simulink model "sampleModel155"  (R2021b)
settings: Solver=VariableStepAuto  StartTime=0.0  StopTime=10.0  RelTol=1e-3
undefined symbols (not defined in the file or in its folder): DiscIntNeverNeededParam, Newton, Raphson
libraries: simulink x4, slpidlib x1
settings Model: Creator=user  LastModifiedBy=user

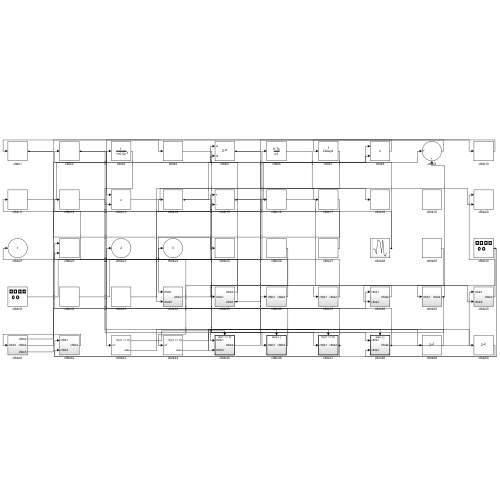
[thumbnail: Simulink's stored preview of the top-level diagram]
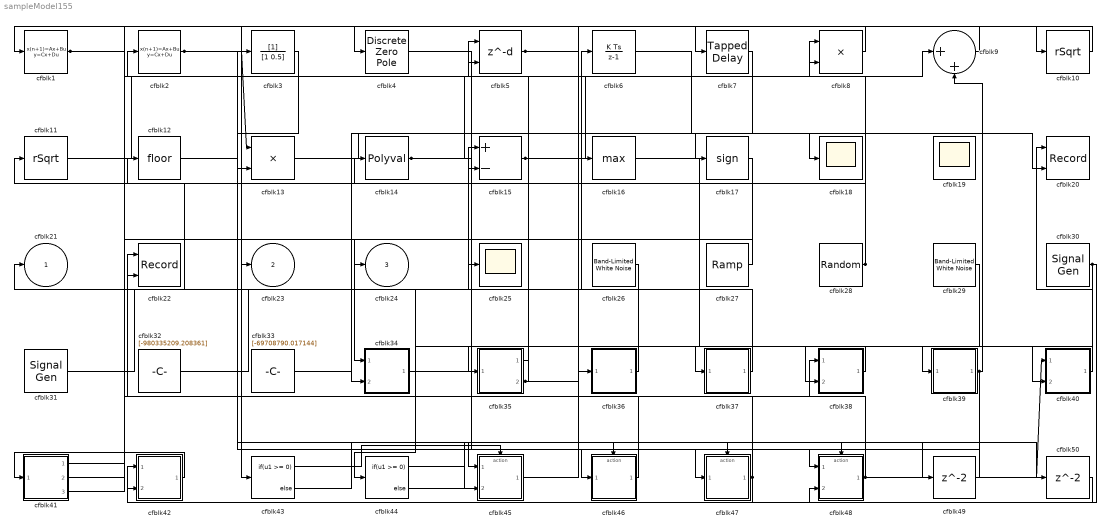
== system sampleModel155 ==
  cfblk1 : DiscreteStateSpace
  cfblk10 : Sqrt  Operator=rSqrt  AlgorithmType=Newton-Raphson  SaturateOnIntegerOverflow=on
  cfblk11 : Sqrt  Operator=rSqrt  AlgorithmType=Newton-Raphson  SaturateOnIntegerOverflow=on
  cfblk12 : Rounding
  cfblk13 : Product  Inputs=**
  cfblk14 : Polyval  Coefs=[ +2.081618890e-019, -1.441693666e-014, +4.719686976e-010, -8.536869453e-006, +1.621573104e-001, -8.087801117e+001 ]
  cfblk15 : Sum  Inputs=+-
  cfblk16 : MinMax  Function=max
  cfblk17 : Signum
  cfblk18 : Scope
  cfblk19 : Scope
      settings: Floating=on
  cfblk2 : DiscreteStateSpace
  cfblk20 : Record  FileSettingsInternal="{\"entries\":[{\"content\":{\"excelSettings\":{\"content\":{},\"type\":\"Streamout.ExcelSettings\"}},\"type\":\"Streamout.FileSettingStorage\",\"uuid\":\"c6a0a69c-cb25-483f-9436-b518442c183b\"}],\"packageUris\":[\"http://schema.mathworks.com/mf0/streamout_blocks/R2020a\"],\"version\":\"1.0\"}"  Layout=[1 1]  SignalsInternal="{\"entries\":[{\"content\":{\"signals\":[{\"content\":{\"blockPath\":[\"sampleModel155/cfblk20\"],\"channel\":[],\"dimensions\":[1],\"domain\":\"sampleModel155/cfblk20\",\"lineColor\":\"#a2142f\",\"plots\":[1],\"port\":1,\"sid\":[\"\"],\"signalID\":5829,\"signalName\":\"cfblk40\"},\"type\":\"RecordBlkView.Signal\",\"uuid\":\"982e78fb-ecc7-4af2-9bce-bf19e89cf4a4\"},{\"content\":{\"blockPath\":[\"sampleModel155/cfblk20\"],\"channel\":[],\"dimensions\":[1],\"domain\":\"sampleModel155/cfblk20\",\"lineColor\":\"#139fff\",\"plots\":[1],\"port\":2,\"sid\":[\"\"],\"signalID\":5833,\"signalName\":\"cfblk6\"},\"type\":\"RecordBlkView.Signal\",\"uuid\":\"4fc80603-e495-4758-b370-e399ca86c921\"}]},\"type\":\"RecordBlkView.InputSignals\",\"uuid\":\"2fc9934d-8013-4f67-99c3-7600cfd9b416\"}],\"packageUris\":[\"http://schema.mathworks.com/mf0/streamout_blocks/R2020a\"],\"version\":\"1.0\"}"  VisualizationBindings="{\"xyplotplugin\":{\"info\":[{\"series\":[{\"bindingParametersList\":[{\"parameter\":\"X-Axis\",\"signalID\":5829,\"signalName\":\"cfblk40\"},{\"parameter\":\"Y-Axis\",\"signalID\":5833,\"signalName\":\"cfblk6\"}],\"seriesID\":42704}],\"subplotID\":1}]}}"  CompatibilityTag=XY
  cfblk22 : Record  FileSettingsInternal="{\"entries\":[{\"content\":{\"excelSettings\":{\"content\":{},\"type\":\"Streamout.ExcelSettings\"}},\"type\":\"Streamout.FileSettingStorage\",\"uuid\":\"4d11d9fd-29c9-4ce8-99ba-2382077eddbc\"}],\"packageUris\":[\"http://schema.mathworks.com/mf0/streamout_blocks/R2020a\"],\"version\":\"1.0\"}"  Layout=[1 1]  SignalsInternal="{\"entries\":[{\"content\":{\"signals\":[{\"content\":{\"blockPath\":[\"sampleModel155/cfblk22\"],\"channel\":[],\"dimensions\":[1],\"domain\":\"sampleModel155/cfblk22\",\"lineColor\":\"#a2142f\",\"plots\":[1],\"port\":1,\"sid\":[\"\"],\"signalID\":5837,\"signalName\":\"cfblk35:2\"},\"type\":\"RecordBlkView.Signal\",\"uuid\":\"607973d4-97f1-4e95-a130-668d98db00e6\"},{\"content\":{\"blockPath\":[\"sampleModel155/cfblk22\"],\"channel\":[],\"dimensions\":[1],\"domain\":\"sampleModel155/cfblk22\",\"lineColor\":\"#139fff\",\"plots\":[1],\"port\":2,\"sid\":[\"\"],\"signalID\":5841,\"signalName\":\"cfblk48\"},\"type\":\"RecordBlkView.Signal\",\"uuid\":\"b323fbb3-43dc-4456-bc21-4a787fbff72d\"}]},\"type\":\"RecordBlkView.InputSignals\",\"uuid\":\"74f477da-4040-45bf-b858-66ad6525a84b\"}],\"packageUris\":[\"http://schema.mathworks.com/mf0/streamout_blocks/R2020a\"],\"version\":\"1.0\"}"  VisualizationBindings="{\"xyplotplugin\":{\"info\":[{\"series\":[{\"bindingParametersList\":[{\"parameter\":\"X-Axis\",\"signalID\":5837,\"signalName\":\"cfblk35:2\"},{\"parameter\":\"Y-Axis\",\"signalID\":5841,\"signalName\":\"cfblk48\"}],\"seriesID\":8769}],\"subplotID\":1}]}}"  CompatibilityTag=XY
  cfblk25 : Scope
  cfblk26 : simulink/Sources/Band-Limited White Noise  Cov=[6682375464.485454]  Ts=0.1  seed=[5360034971.000000]
  cfblk27 : simulink/Sources/Ramp  slope=[-7060.642561]  start=[21.976533]  InitialOutput=[864381.445498]
  cfblk28 : RandomNumber  Mean=[-62257.725679]  Variance=[20771.732840]  Seed=[583175511.000000]  SampleTime=0.1
  cfblk29 : simulink/Sources/Band-Limited White Noise  Cov=[2781141721.159909]  Ts=0.1  seed=[7793621344.000000]
  cfblk3 : DiscreteFilter  SampleTime=1
  cfblk30 : SignalGenerator  Amplitude=[-532353384.064106]
  cfblk31 : SignalGenerator  WaveForm=sawtooth  Amplitude=[-996285201.899179]  Units=rad/sec
  cfblk32 : Constant  Value=[-980335209.208361]  SampleTime=1
  cfblk33 : Constant  Value=[-69708790.017144]  SampleTime=1
  cfblk34 : Subsystem
  cfblk35 : Subsystem
  cfblk36 : Subsystem
  cfblk37 : Subsystem
  cfblk38 : Subsystem
  cfblk39 : Subsystem
  cfblk4 : DiscreteZeroPole  Poles=[0 0.5]  Gain=1
  cfblk40 : Subsystem
  cfblk41 : Subsystem
  cfblk42 : Subsystem
  cfblk43 : If  IfExpression=u1 >= 0  SampleTime=1
  cfblk44 : If  IfExpression=u1 >= 0  SampleTime=1
  cfblk45 : Subsystem  TreatAsAtomicUnit=on
  cfblk46 : Subsystem  TreatAsAtomicUnit=on
  cfblk47 : Subsystem  TreatAsAtomicUnit=on
  cfblk48 : Subsystem  TreatAsAtomicUnit=on
  cfblk49 : Delay  SampleTime=1
  cfblk5 : Delay  DelayLengthSource=Input port  SampleTime=1
      settings: InputPortMap=u0,p1
  cfblk50 : Delay  SampleTime=1
  cfblk6 : DiscreteIntegrator  ICPrevOutput=DiscIntNeverNeededParam  ICPrevScaledInput=DiscIntNeverNeededParam
  cfblk7 : simulink/Discrete/Tapped Delay  vinit=0.0  samptime=-1  NumDelays=1  DelayOrder=Oldest  includeCurrent=off
  cfblk8 : Product
  cfblk9 : Sum  Inputs=|++
  cfblk21 : Outport
  cfblk23 : Outport  Port=2
  cfblk24 : Outport  Port=3
  wires:
  cfblk4/1 -> cfblk48/1(cfblk1)
  cfblk48/1(cfblk2) -> cfblk40/1(cfblk1), cfblk22/2
  cfblk17/1 -> cfblk34/1(cfblk1)
  cfblk14/1 -> cfblk46/1(cfblk1), cfblk8/2
  cfblk10/1 -> cfblk43/1
  cfblk27/1 -> cfblk11/1
  cfblk29/1 -> cfblk39/1(cfblk1)
  cfblk32/1 -> cfblk15/1
  cfblk28/1 -> cfblk2/1, cfblk14/1
  cfblk45/1(cfblk2) -> cfblk36/1(cfblk1)
  cfblk13/1 -> cfblk18/1
  cfblk34/1(cfblk2) -> cfblk37/1(cfblk1)
  cfblk30/1 -> cfblk42/1(cfblk1), cfblk38/2(cfblk4)
  cfblk26/1 -> cfblk44/1
  cfblk2/1 -> cfblk13/1, cfblk47/1(cfblk1)
  cfblk41/1(cfblk2) -> cfblk5/1
  cfblk46/1(cfblk2) -> cfblk23/1
  cfblk1/1 -> cfblk25/1, cfblk4/1
  cfblk40/1(cfblk2) -> cfblk20/1
  cfblk9/1 -> cfblk7/1
  cfblk6/1 -> cfblk20/2
  cfblk7/1 -> cfblk34/2(cfblk3)
  cfblk31/1 -> cfblk6/1
  cfblk42/1(cfblk2) -> cfblk41/1(cfblk1)
  cfblk3/1 -> cfblk13/2
  cfblk39/1(cfblk2) -> cfblk45/2(cfblk5), cfblk9/2
  cfblk47/1(cfblk2) -> cfblk24/1, cfblk42/2(cfblk3)
  cfblk41/2(cfblk4) -> cfblk38/1(cfblk1)
  cfblk8/1 -> cfblk1/1
  cfblk15/1 -> cfblk9/1, cfblk50/1
  cfblk38/1(cfblk2) -> cfblk35/1(cfblk1)
  cfblk35/1(cfblk2) -> cfblk5/2
  cfblk16/1 -> cfblk40/2(cfblk5)
  cfblk5/1 -> cfblk10/1, cfblk17/1
  cfblk37/1(cfblk2) -> cfblk21/1
  cfblk11/1 -> cfblk3/1
  cfblk35/2(cfblk3) -> cfblk22/1, cfblk8/1
  cfblk41/3(cfblk5) -> cfblk15/2
  cfblk36/1(cfblk2) -> cfblk12/1
  cfblk33/1 -> cfblk16/1
  cfblk43/1 -> cfblk45/Action
  cfblk43/2 -> cfblk46/Action
  cfblk44/1 -> cfblk47/Action
  cfblk44/2 -> cfblk48/Action
  cfblk12/1 -> cfblk49/1
  cfblk49/1 -> cfblk45/1(cfblk1)
  cfblk50/1 -> cfblk48/2(cfblk4)

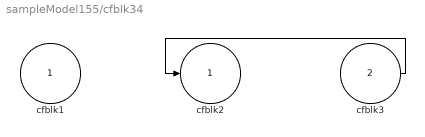
== system sampleModel155/cfblk34 ==
  cfblk1 : Inport
  cfblk3 : Inport  Port=2
  cfblk2 : Outport
  wires:
  cfblk3/1 -> cfblk2/1

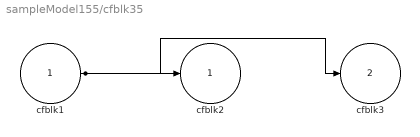
== system sampleModel155/cfblk35 ==
  cfblk1 : Inport
  cfblk2 : Outport
  cfblk3 : Outport  Port=2
  wires:
  cfblk1/1 -> cfblk2/1, cfblk3/1

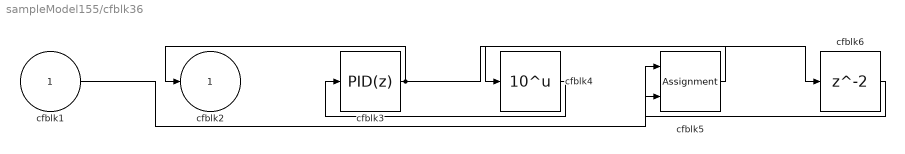
== system sampleModel155/cfblk36 ==
  cfblk1 : Inport
  cfblk3 : slpidlib/PID Controller  Controller=PID  Form=Parallel  TimeDomain=Discrete-time  UseExternalTs=off  SampleTime=1  IntegratorMethod=Forward Euler  FilterMethod=Forward Euler  ControllerParametersSource=internal  P=1  I=1  D=0  UseFilter=on  N=100  TunerSelectOption=Transfer Function Based (PID Tuner App)  InitialConditionSource=internal  InitialConditionForIntegrator=0  InitialConditionForFilter=0  DifferentiatorICPrevScaledInput=0  ExternalReset=none  TrackingMode=off  Kt=1  LimitOutput=off  SatLimitsSource=internal  UpperSaturationLimit=inf  LowerSaturationLimit=-inf  LinearizeAsGain=off  AntiWindupMode=none  Kb=1  POutMin=[]  POutMax=[]  IOutMin=[]  IOutMax=[]  DOutMin=[]  DOutMax=[]  NOutMin=[]  NOutMax=[]  SumOutMin=[]  SumOutMax=[]  SaturationOutMin=[]  SaturationOutMax=[]  PParamMin=[]  PParamMax=[]  IParamMin=[]  IParamMax=[]  DParamMin=[]  DParamMax=[]  NParamMin=[]  NParamMax=[]  KbParamMin=[]  KbParamMax=[]  KtParamMin=[]  KtParamMax=[]  KbOutMin=[]  KbOutMax=[]  KtOutMin=[]  KtOutMax=[]  IntegratorOutMin=[]  IntegratorOutMax=[]  FilterOutMin=[]  FilterOutMax=[]  SumI1OutMin=[]  SumI1OutMax=[]  SumI2OutMin=[]  SumI2OutMax=[]  SumI3OutMin=[]  SumI3OutMax=[]  SumI4OutMin=[]  SumI4OutMax=[]  SumDOutMin=[]  SumDOutMax=[]  DifferentiatorOutMin=[]  DifferentiatorOutMax=[]  FilterDiffOutCoefMin=[]  FilterDiffOutCoefMax=[]  ReciprocalOutMin=[]  ReciprocalOutMax=[]  SumDenOutMin=[]  SumDenOutMax=[]  SumNumOutMin=[]  SumNumOutMax=[]  DivideOutMin=[]  DivideOutMax=[]  UdiffTsProdOutMin=[]  UdiffTsProdOutMax=[]  NTsProdOutMin=[]  NTsProdOutMax=[]  UintegralTsProdOutMin=[]  UintegralTsProdOutMax=[]  UngainTsProdOutMin=[]  UngainTsProdOutMax=[]  IntegratorContinuousStateAttributes=''  IntegratorStateMustResolveToSignalObject=off  IntegratorRTWStateStorageClass=Auto  FilterContinuousStateAttributes=''  FilterStateMustResolveToSignalObject=off  FilterRTWStateStorageClass=Auto  ParallelPVariant=InternalParameters  IdealPVariant=Disabled  IVariant=InternalParameters  DVariant=InternalParameters  IntegratorVariant=Discrete  SatVariant=Disabled  AWVariant=Passthrough  PCopyVariant=Disabled  TRVariant=Disabled  FdbkBlocksVariant=Forward  IdealPFdbkVariant=Disabled  SatFdbkVariant=Disabled  DerivativeFilterVariant=ForwardEulerFilter  NVariant=InternalParameters  NCopyVariant=Disabled  FilterICVariant=InternalICsFilter  IntegratorICVariant=InternalICs  ExternalResetVariant=Disabled  TRSumVariant=Passthrough  SumFdbkVariant=Disabled  SumVariant=Sum_PID  TsampFilterVariant=InternalTs  TsampNgainVariant=Passthrough  TsampIntegralVariant=Passthrough  ExternalSaturationOutDataTypeStr=Inherit: Same as second input
  cfblk4 : Math  Operator=10^u  SaturateOnIntegerOverflow=on
  cfblk5 : Assignment  DiagnosticForDimensions=Warning  IndexOptions=Index vector (dialog)  Indices=1  OutputSizes=1
  cfblk6 : Delay  SampleTime=1
  cfblk2 : Outport
  wires:
  cfblk3/1 -> cfblk2/1, cfblk6/1
  cfblk5/1 -> cfblk4/1
  cfblk4/1 -> cfblk3/1
  cfblk1/1 -> cfblk5/1
  cfblk6/1 -> cfblk5/2

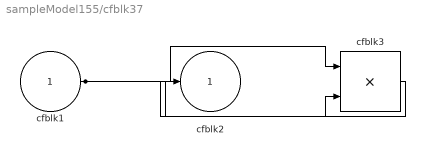
== system sampleModel155/cfblk37 ==
  cfblk1 : Inport
  cfblk3 : Product  Inputs=**
  cfblk2 : Outport
  wires:
  cfblk1/1 -> cfblk3/1, cfblk3/2
  cfblk3/1 -> cfblk2/1

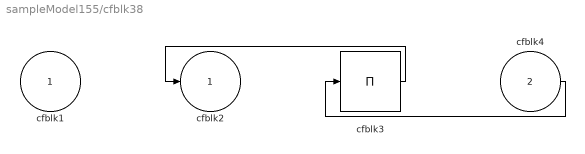
== system sampleModel155/cfblk38 ==
  cfblk1 : Inport
  cfblk4 : Inport  Port=2
  cfblk3 : Product  Inputs=*
  cfblk2 : Outport
  wires:
  cfblk3/1 -> cfblk2/1
  cfblk4/1 -> cfblk3/1

== system sampleModel155/cfblk39 ==
  cfblk1 : Inport
  cfblk3 : Rounding
  cfblk2 : Outport
  wires:
  cfblk1/1 -> cfblk3/1
  cfblk3/1 -> cfblk2/1

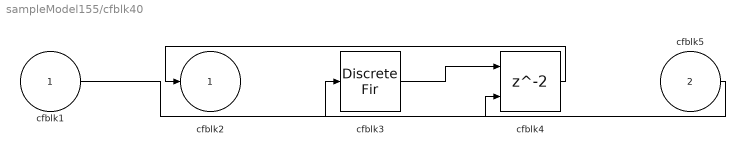
== system sampleModel155/cfblk40 ==
  cfblk1 : Inport
  cfblk5 : Inport  Port=2
  cfblk3 : DiscreteFir  SampleTime=1
  cfblk4 : Delay  ShowEnablePort=on  SampleTime=1
      settings: InputPortMap=u0,e6
  cfblk2 : Outport
  wires:
  cfblk4/1 -> cfblk2/1
  cfblk3/1 -> cfblk4/1
  cfblk5/1 -> cfblk3/1
  cfblk1/1 -> cfblk4/2

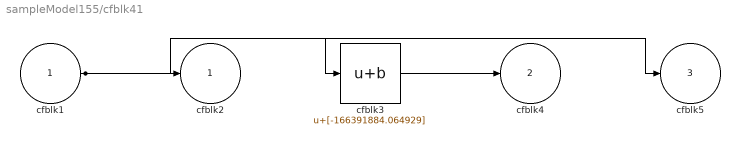
== system sampleModel155/cfblk41 ==
  cfblk1 : Inport
  cfblk3 : Bias  Bias=[-166391884.064929]
  cfblk2 : Outport
  cfblk4 : Outport  Port=2
  cfblk5 : Outport  Port=3
  wires:
  cfblk3/1 -> cfblk4/1
  cfblk1/1 -> cfblk3/1, cfblk5/1, cfblk2/1

== system sampleModel155/cfblk42 ==
  cfblk1 : Inport
  cfblk3 : Inport  Port=2
  cfblk2 : Outport
  wires:
  cfblk1/1 -> cfblk2/1

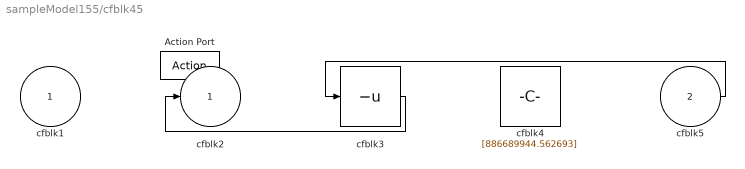
== system sampleModel155/cfblk45 ==
  cfblk1 : Inport
  cfblk5 : Inport  Port=2
  Action Port : ActionPort  ActionPortLabel=if(u1 >= 0)
  cfblk3 : UnaryMinus
  cfblk4 : Constant  Value=[886689944.562693]  SampleTime=1
  cfblk2 : Outport
  wires:
  cfblk3/1 -> cfblk2/1
  cfblk5/1 -> cfblk3/1

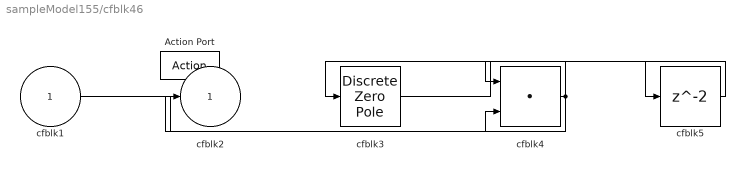
== system sampleModel155/cfblk46 ==
  cfblk1 : Inport
  Action Port : ActionPort  ActionPortLabel=else
  cfblk3 : DiscreteZeroPole  Poles=[0 0.5]  Gain=1  SampleTime=-1
  cfblk4 : DotProduct  InputSameDT=on  OutDataTypeStr=Inherit: Inherit via internal rule
  cfblk5 : Delay
  cfblk2 : Outport
  wires:
  cfblk1/1 -> cfblk4/2
  cfblk4/1 -> cfblk3/1, cfblk2/1
  cfblk3/1 -> cfblk5/1
  cfblk5/1 -> cfblk4/1

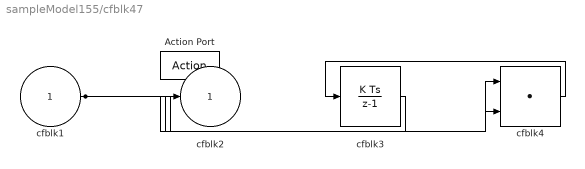
== system sampleModel155/cfblk47 ==
  cfblk1 : Inport
  Action Port : ActionPort  ActionPortLabel=if(u1 >= 0)
  cfblk3 : DiscreteIntegrator  SampleTime=-1  ICPrevOutput=DiscIntNeverNeededParam  ICPrevScaledInput=DiscIntNeverNeededParam
  cfblk4 : DotProduct  InputSameDT=on  OutDataTypeStr=Inherit: Inherit via internal rule
  cfblk2 : Outport
  wires:
  cfblk1/1 -> cfblk4/1, cfblk4/2
  cfblk4/1 -> cfblk3/1
  cfblk3/1 -> cfblk2/1

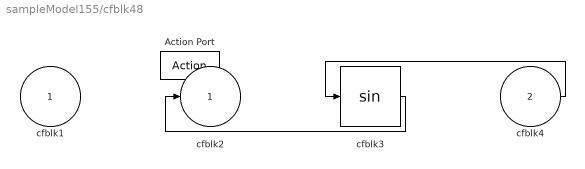
== system sampleModel155/cfblk48 ==
  cfblk1 : Inport
  cfblk4 : Inport  Port=2
  Action Port : ActionPort  ActionPortLabel=else
  cfblk3 : Trigonometry
  cfblk2 : Outport
  wires:
  cfblk3/1 -> cfblk2/1
  cfblk4/1 -> cfblk3/1
